simulink model "RmsConverterController_AAvdM_R2014b"  (R2014b)
settings: Solver=ode45  StartTime=0.0  StopTime=10.0  FixedStep=1e-3  RelTol=1e-3
libraries: simulink x5
settings Model: Creator=sandroni  LastModifiedBy=Arjen
settings DataIOCC: LimitDataPoints=off  SaveFormat=StructureWithTime
settings OptimizationCC: UseDivisionForNetSlopeComputation=off  SimCompilerOptimization=off
settings DebuggingCC: SolverPrmCheckMsg=none  FcnCallInpInsideContextMsg=error  FrameProcessingCompatibilityMsg=error  SFUnexpectedBacktrackingDiag=error  SFNoUnconditionalDefaultTransitionDiag=error  SFExecutionAtInitializationDiag=none
settings HardwareCC: ProdBitPerPointer=64  ProdBitPerSizeT=32  ProdBitPerPtrDiffT=32  ProdLargestAtomicFloat=Float  ProdIntDivRoundTo=Zero  ProdEndianess=LittleEndian  ProdHWDeviceType=Specified  TargetBitPerPointer=64  TargetBitPerSizeT=64  TargetBitPerPtrDiffT=64  TargetLongLongMode=on  TargetIntDivRoundTo=Zero  TargetEndianess=LittleEndian  TargetWordSize=64  TargetHWDeviceType=MATLAB Host  ProdEqTarget=off
settings ModelReferenceCC: PropagateSignalLabelsOutOfModel=on
settings RTWCC: SystemTargetFile=rtwsfcnfmi.tlc  TemplateMakefile=rtwsfcnfmi_tmf  Description=S-Function Target with Functional Mockup Interface (FMI)  RTWCompilerOptimization=off
settings STFCustomTargetCC: ModelReferenceCompliant=off  CompOptLevelCompliant=on  GeneratePreprocessorConditionals=Disable all  MATLABClassNameForMDSCustomization=Simulink.SoftwareTarget.TargetSpecificTriggerConfigurationBase  SystemTargetFile=rtwsfcnfmi.tlc
settings ConfigurationSet: Description=Simscape Multibody

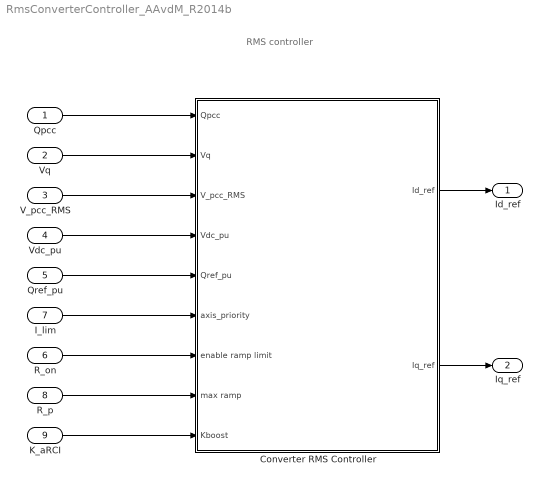
== system RmsConverterController_AAvdM_R2014b ==
  note: RMS controller
  Qpcc : Inport
  Vq : Inport  Port=2
  V_pcc_RMS : Inport  Port=3
  Vdc_pu : Inport  Port=4
  Qref_pu : Inport  Port=5
  R_on : Inport  Port=6
  I_lim : Inport  Port=7
  R_p : Inport  Port=8
  K_aRCI : Inport  Port=9
  Converter RMS Controller : Subsystem  mask(Converter RMS Controller){Kp_dc=1.1, Ki_dc=27.5, Kp_Var=1, Ki_Var=100, P0_pu=0.85, Fnom=50, Ts=2e-5, RP=1, Imax_grid_conv=1.1}
      mask prompts: Kp_dc "DC voltage regulator proportional parameter [Kp]"; Ki_dc "DC voltage regulator integral parameter [Ki]"; Kp_Var "PCC voltage regulator proportional parameter [Kp]"; Ki_Var "PCC voltage regulator integral parameter [Ki]"; P0_pu "Initial Active Power [pu]"; Fnom "Nominal frequency [Hz]"; Ts "Sample Time [s]"; RP "max ramp rate [pu/s]"; Imax_grid_conv "overcurrent limit [pu]"
  Id_ref : Outport
  Iq_ref : Outport  Port=2
  wires:
  Qref_pu/1 -> Converter RMS Controller/5(Qref_pu)
  V_pcc_RMS/1 -> Converter RMS Controller/3(V_pcc_RMS)
  K_aRCI/1 -> Converter RMS Controller/9(Kboost)
  R_p/1 -> Converter RMS Controller/8(max ramp)
  Converter RMS Controller/1(Id_ref) -> Id_ref/1
  Converter RMS Controller/2(Iq_ref) -> Iq_ref/1
  Vq/1 -> Converter RMS Controller/2(Vq)
  Vdc_pu/1 -> Converter RMS Controller/4(Vdc_pu)
  Qpcc/1 -> Converter RMS Controller/1(Qpcc)
  R_on/1 -> Converter RMS Controller/7(enable ramp limit)
  I_lim/1 -> Converter RMS Controller/6(axis_priority)

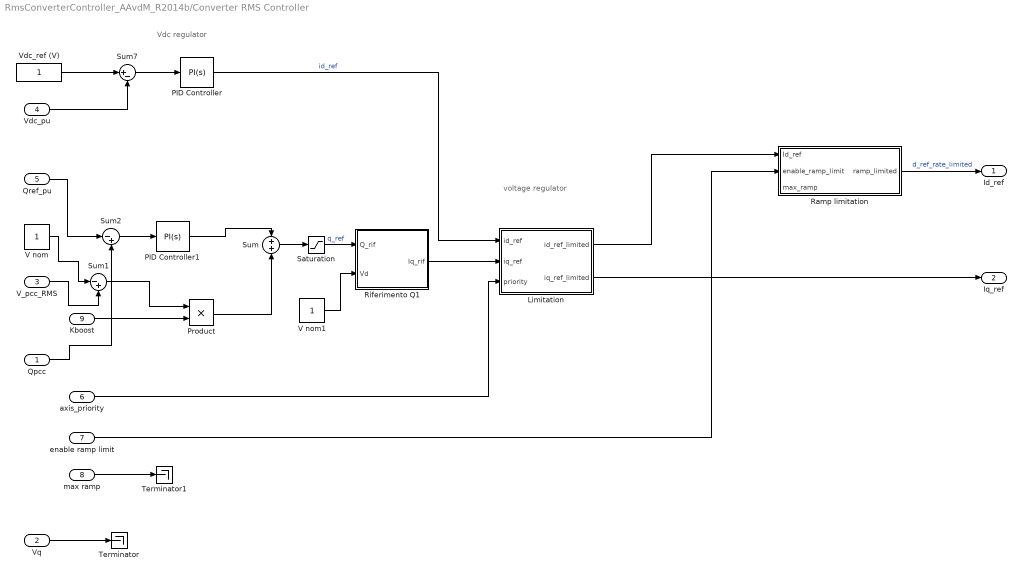
== system RmsConverterController_AAvdM_R2014b/Converter RMS Controller ==
  note: Vdc regulator
  note: voltage regulator
  Qpcc : Inport
  Vq : Inport  Port=2
  V_pcc_RMS : Inport  Port=3
  Vdc_pu : Inport  Port=4
  Qref_pu : Inport  Port=5
  axis_priority : Inport  Port=6
  enable ramp limit : Inport  Port=7
  max ramp : Inport  Port=8
  Kboost : Inport  Port=9
  Limitation : Subsystem
  PID Controller : simulink/Continuous/PID Controller  Controller=PI  TimeDomain=Continuous-time  SampleTime=-1  IntegratorMethod=Forward Euler  FilterMethod=Forward Euler  Form=Parallel  P=1  I=1  D=0  N=100  InitialConditionSource=internal  InitialConditionForIntegrator=0  InitialConditionForFilter=0  ExternalReset=none  LimitOutput=on  UpperSaturationLimit=inf  LowerSaturationLimit=-inf  LinearizeAsGain=on  AntiWindupMode=none  Kb=1  TrackingMode=off  Kt=1  PParamMin=[]  PParamMax=[]  IParamMin=[]  IParamMax=[]  DParamMin=[]  DParamMax=[]  NParamMin=[]  NParamMax=[]  KbParamMin=[]  KbParamMax=[]  KtParamMin=[]  KtParamMax=[]  POutMin=[]  POutMax=[]  IOutMin=[]  IOutMax=[]  DOutMin=[]  DOutMax=[]  NOutMin=[]  NOutMax=[]  KbOutMin=[]  KbOutMax=[]  KtOutMin=[]  KtOutMax=[]  IntegratorOutMin=[]  IntegratorOutMax=[]  FilterOutMin=[]  FilterOutMax=[]  SumOutMin=[]  SumOutMax=[]  SumI1OutMin=[]  SumI1OutMax=[]  SumI2OutMin=[]  SumI2OutMax=[]  SumI3OutMin=[]  SumI3OutMax=[]  SumDOutMin=[]  SumDOutMax=[]  SaturationOutMin=[]  SaturationOutMax=[]  IntegratorContinuousStateAttributes=''  IntegratorStateMustResolveToSignalObject=off  IntegratorRTWStateStorageClass=Auto  FilterContinuousStateAttributes=''  FilterStateMustResolveToSignalObject=off  FilterRTWStateStorageClass=Auto  DifferentiatorICPrevScaledInput=0  DifferentiatorOutMin=[]  DifferentiatorOutMax=[]  UseFilter=on
  PID Controller1 : simulink/Continuous/PID Controller  Controller=PI  TimeDomain=Continuous-time  SampleTime=-1  IntegratorMethod=Forward Euler  FilterMethod=Forward Euler  Form=Parallel  P=1  I=1  D=0  N=100  InitialConditionSource=internal  InitialConditionForIntegrator=0  InitialConditionForFilter=0  ExternalReset=none  LimitOutput=on  UpperSaturationLimit=inf  LowerSaturationLimit=-inf  LinearizeAsGain=on  AntiWindupMode=none  Kb=1  TrackingMode=off  Kt=1  PParamMin=[]  PParamMax=[]  IParamMin=[]  IParamMax=[]  DParamMin=[]  DParamMax=[]  NParamMin=[]  NParamMax=[]  KbParamMin=[]  KbParamMax=[]  KtParamMin=[]  KtParamMax=[]  POutMin=[]  POutMax=[]  IOutMin=[]  IOutMax=[]  DOutMin=[]  DOutMax=[]  NOutMin=[]  NOutMax=[]  KbOutMin=[]  KbOutMax=[]  KtOutMin=[]  KtOutMax=[]  IntegratorOutMin=[]  IntegratorOutMax=[]  FilterOutMin=[]  FilterOutMax=[]  SumOutMin=[]  SumOutMax=[]  SumI1OutMin=[]  SumI1OutMax=[]  SumI2OutMin=[]  SumI2OutMax=[]  SumI3OutMin=[]  SumI3OutMax=[]  SumDOutMin=[]  SumDOutMax=[]  SaturationOutMin=[]  SaturationOutMax=[]  IntegratorContinuousStateAttributes=''  IntegratorStateMustResolveToSignalObject=off  IntegratorRTWStateStorageClass=Auto  FilterContinuousStateAttributes=''  FilterStateMustResolveToSignalObject=off  FilterRTWStateStorageClass=Auto  DifferentiatorICPrevScaledInput=0  DifferentiatorOutMin=[]  DifferentiatorOutMax=[]  UseFilter=on
  Product : Product
  Ramp limitation : Subsystem
  Riferimento Q1 : Subsystem
  Saturation : Saturate  UpperLimit=Imax_grid_conv  LowerLimit=-Imax_grid_conv
  Sum : Sum
  Sum1 : Sum  Inputs=|-+  SaturateOnIntegerOverflow=on  InputSameDT=on  OutDataTypeStr=Inherit: Same as first input
  Sum2 : Sum  Inputs=|-+  SaturateOnIntegerOverflow=on  InputSameDT=on  OutDataTypeStr=Inherit: Same as first input
  Sum7 : Sum  Inputs=|+-  SaturateOnIntegerOverflow=on  InputSameDT=on  OutDataTypeStr=Inherit: Same as first input
  Terminator : Terminator
  Terminator1 : Terminator
  V nom : Constant
  V nom1 : Constant
  Vdc_ref (V) : Constant
  Id_ref : Outport
  Iq_ref : Outport  Port=2
  wires:
  Vdc_ref (V)/1 -> Sum7/1
  Qpcc/1 -> Sum2/2
  Qref_pu/1 -> Sum2/1
  Sum/1 -> Saturation/1
  Saturation/1 -> Riferimento Q1/1(Q_rif)  "q_ref"
  Vdc_pu/1 -> Sum7/2
  axis_priority/1 -> Limitation/3(priority)
  Riferimento Q1/1(Iq_rif) -> Limitation/2(iq_ref)
  PID Controller/1 -> Limitation/1(id_ref)  "id_ref"
  Limitation/2(iq_ref_limited) -> Iq_ref/1
  Ramp limitation/1(ramp_limited) -> Id_ref/1  "d_ref_rate_limited"
  Limitation/1(id_ref_limited) -> Ramp limitation/1(Id_ref)
  enable ramp limit/1 -> Ramp limitation/2(enable_ramp_limit)
  Vq/1 -> Terminator/1
  Sum7/1 -> PID Controller/1
  Sum2/1 -> PID Controller1/1
  Kboost/1 -> Product/2
  max ramp/1 -> Terminator1/1
  V nom1/1 -> Riferimento Q1/2(Vd)
  V nom/1 -> Sum1/1
  V_pcc_RMS/1 -> Sum1/2
  Sum1/1 -> Product/1
  PID Controller1/1 -> Sum/1
  Product/1 -> Sum/2

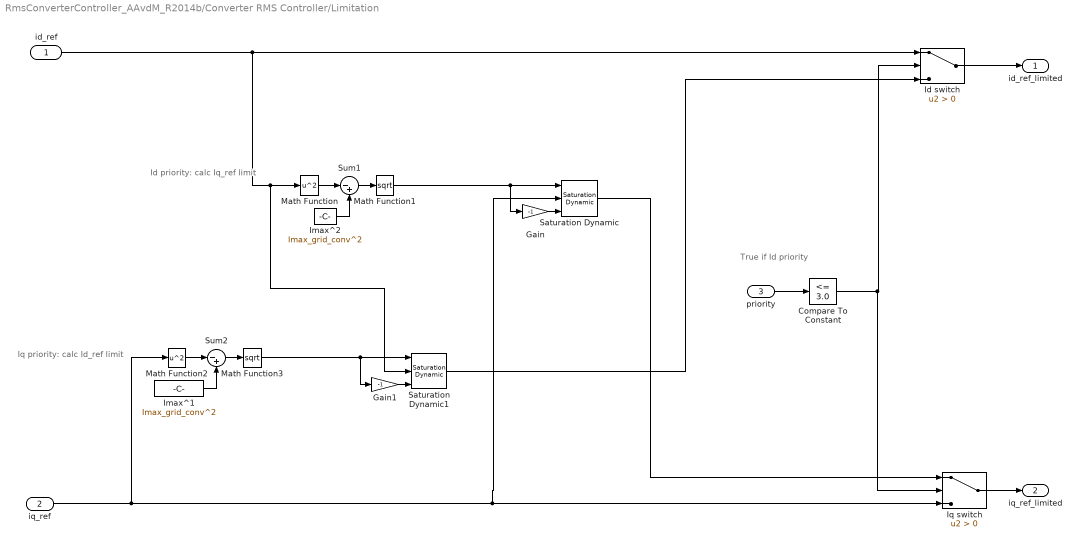
== system RmsConverterController_AAvdM_R2014b/Converter RMS Controller/Limitation ==
  note: Id priority:
      | calc Iq_ref limit
  note: True if Id priority
  note: Iq priority:
      | calc Id_ref limit
  id_ref : Inport
  iq_ref : Inport  Port=2
  priority : Inport  Port=3
  Compare To Constant : simulink/Logic and Bit Operations/Compare To Constant  relop=<=  const=3.0  OutDataTypeStr=boolean
  Gain : Gain  Gain=-1
  Gain1 : Gain  Gain=-1
  Id switch : Switch  Criteria=u2 > Threshold
  Imax^1 : Constant  Value=Imax_grid_conv^2
  Imax^2 : Constant  Value=Imax_grid_conv^2
  Iq switch : Switch  Criteria=u2 > Threshold
  Math Function : Math  Operator=square  SaturateOnIntegerOverflow=on
  Math Function1 : Math  Operator=sqrt  SaturateOnIntegerOverflow=on
  Math Function2 : Math  Operator=square  SaturateOnIntegerOverflow=on
  Math Function3 : Math  Operator=sqrt  SaturateOnIntegerOverflow=on
  Saturation Dynamic : simulink/Discontinuities/Saturation Dynamic  OutMin=[]  OutMax=[]  OutDataTypeStr=Inherit: Same as second input  OutDataType=fixdt(1, 16)  OutScaling=2^-10  DoSatur=off
  Saturation Dynamic1 : simulink/Discontinuities/Saturation Dynamic  OutMin=[]  OutMax=[]  OutDataTypeStr=Inherit: Same as second input  OutDataType=fixdt(1, 16)  OutScaling=2^-10  DoSatur=off
  Sum1 : Sum  Inputs=|-+  SaturateOnIntegerOverflow=on  InputSameDT=on  OutDataTypeStr=Inherit: Same as first input
  Sum2 : Sum  Inputs=|-+  SaturateOnIntegerOverflow=on  InputSameDT=on  OutDataTypeStr=Inherit: Same as first input
  id_ref_limited : Outport
  iq_ref_limited : Outport  Port=2
  wires:
  Imax^2/1 -> Sum1/2
  Math Function/1 -> Sum1/1
  Sum1/1 -> Math Function1/1
  Gain/1 -> Saturation Dynamic/3
  priority/1 -> Compare To Constant/1
  Compare To Constant/1 -> Iq switch/2, Id switch/2
  Saturation Dynamic/1 -> Iq switch/1
  Imax^1/1 -> Sum2/2
  Math Function2/1 -> Sum2/1
  Sum2/1 -> Math Function3/1
  Gain1/1 -> Saturation Dynamic1/3
  Saturation Dynamic1/1 -> Id switch/3
  Id switch/1 -> id_ref_limited/1
  Iq switch/1 -> iq_ref_limited/1
  id_ref/1 -> Saturation Dynamic1/2, Math Function/1, Id switch/1
  iq_ref/1 -> Math Function2/1, Saturation Dynamic/2, Iq switch/3
  Math Function1/1 -> Gain/1, Saturation Dynamic/1
  Math Function3/1 -> Gain1/1, Saturation Dynamic1/1

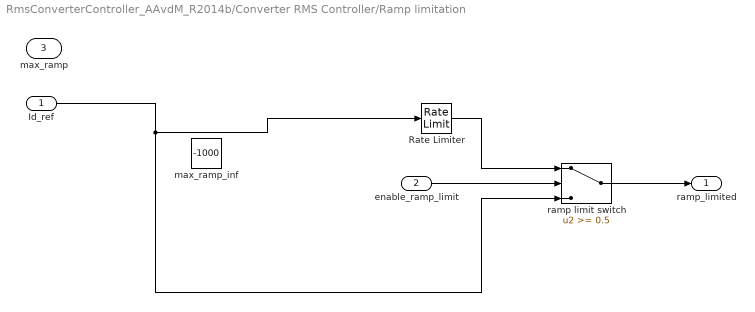
== system RmsConverterController_AAvdM_R2014b/Converter RMS Controller/Ramp limitation ==
  Id_ref : Inport
  enable_ramp_limit : Inport  Port=2
  max_ramp : Inport  Port=3
  Rate Limiter : RateLimiter  RisingSlewLimit=RP  FallingSlewLimit=-1000  SampleTimeMode=inherited
  max_ramp_inf : Constant  Value=-1000
  ramp limit switch : Switch  Threshold=0.5
  ramp_limited : Outport
  wires:
  ramp limit switch/1 -> ramp_limited/1
  Id_ref/1 -> Rate Limiter/1, ramp limit switch/3
  enable_ramp_limit/1 -> ramp limit switch/2
  Rate Limiter/1 -> ramp limit switch/1

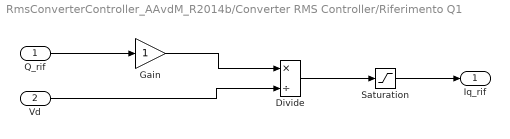
== system RmsConverterController_AAvdM_R2014b/Converter RMS Controller/Riferimento Q1 ==
  Q_rif : Inport
  Vd : Inport  Port=2
  Divide : Product  Inputs=*/
  Gain : Gain
  Saturation : Saturate  UpperLimit=Imax_grid_conv  LowerLimit=-Imax_grid_conv
  Iq_rif : Outport
  wires:
  Vd/1 -> Divide/2
  Gain/1 -> Divide/1
  Q_rif/1 -> Gain/1
  Divide/1 -> Saturation/1
  Saturation/1 -> Iq_rif/1
